simulink model "kenONpart2"  (R2024a)
settings: Solver=VariableStepAuto  StartTime=0.0  StopTime=10.0  RelTol=1e-3
settings Model: Creator=coope  LastModifiedBy=coope

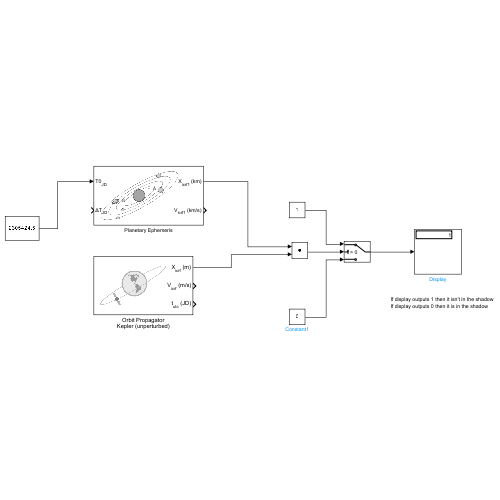
[thumbnail: Simulink's stored preview of the top-level diagram]
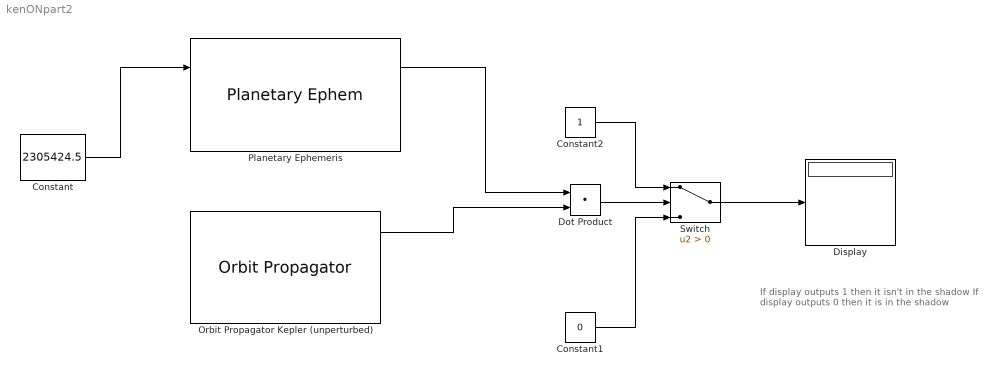
== system kenONpart2 ==
  note: If display outputs 1 then it isn't in the shadow
      | If display outputs 0 then it is in the shadow
  Constant : Constant  Value=2305424.5
  Constant1 : Constant  Value=0
  Constant2 : Constant
  Display : Display
  Dot Product : DotProduct  OutDataTypeStr=Inherit: Inherit via internal rule
  Orbit Propagator Kepler (unperturbed) : OrbitPropagator  inclination=0  inertialPosition=[3649700.0 3308200.0 -4676600.0]  inertialVelocity=[-2750.8 6666.4 2573.4]  fixedPosition=[-4142689.0 -2676864.7 -4669861.6]  fixedVelocity=[1452.7 -6720.7 2568.1]  customR=3396200  customMu=4.305e13  customJ2=1.0826269e-03  customOmega=4.06125949e-3
  Planetary Ephemeris : PlanetaryEphem  epochFormat=T0 and elapsed Julian time  center=Sun  target=Earth
  Switch : Switch  Criteria=u2 > Threshold  SaturateOnIntegerOverflow=off  InputSameDT=off
  wires:
  Orbit Propagator Kepler (unperturbed)/1 -> Dot Product/2
  Planetary Ephemeris/1 -> Dot Product/1
  Constant/1 -> Planetary Ephemeris/1
  Constant1/1 -> Switch/3
  Dot Product/1 -> Switch/2
  Constant2/1 -> Switch/1
  Switch/1 -> Display/1
